simulink model "deadbeat cotroller"  (R2018b)
settings: Solver=VariableStepAuto  StartTime=0.0  StopTime=100  RelTol=1e-3
undefined symbols (not defined in the file or in its folder): den, num
settings Model: Creator=Asus  LastModifiedBy=Asus

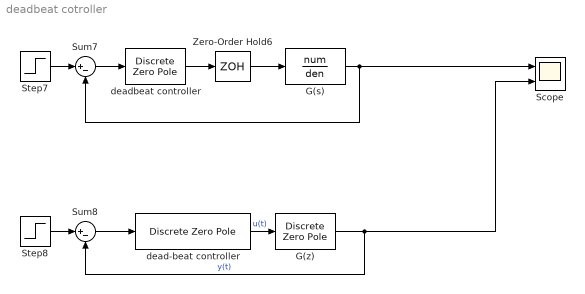
== system deadbeat cotroller ==
  G(s) : TransferFcn  Numerator=num  Denominator=den
  G(z) : DiscreteZeroPole  Zeros="[-2.905  -0.2032]"  Poles="[1  0.7985 0.4356]"  Gain=-0.00046  SampleTime=9
  Scope : Scope  NumInputPorts=2
  Step7 : Step  Time=0  SampleTime=0
  Step8 : Step  Time=0  SampleTime=0
  Sum7 : Sum  Inputs=|+-
  Sum8 : Sum  Inputs=|+-
  Zero-Order Hold6 : ZeroOrderHold  SampleTime=9
  dead-beat controller : DiscreteZeroPole  Zeros=[0.7985 0.4356]  Poles=[-0.5647 -0.2225]  Gain=-0.2128/0.00046  SampleTime=9
  "deadbeat controller " : DiscreteZeroPole  Zeros=[0.7985 0.4356]  Poles=[-0.5647 -0.2225]  Gain=-0.2128/0.00046  SampleTime=9
  wires:
  "deadbeat controller "/1 -> Zero-Order Hold6/1
  Sum7/1 -> "deadbeat controller "/1
  Step8/1 -> Sum8/1
  Step7/1 -> Sum7/1
  G(s)/1 -> Sum7/2, Scope/1
  Sum8/1 -> dead-beat controller/1
  dead-beat controller/1 -> G(z)/1  "u(t)"
  G(z)/1 -> Scope/2, Sum8/2  "y(t)"
  Zero-Order Hold6/1 -> G(s)/1
